simulink library "INT_ASDrf_SelectParameter"  (R2016b)
settings: Solver=VariableStepAuto  StartTime=0.0  StopTime=10.0  RelTol=1e-3
settings Model: Creator=lenovo  LastModifiedBy=lenovo

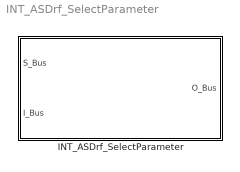
== system INT_ASDrf_SelectParameter ==
  INT_ASDrf_SelectParameter : Subsystem

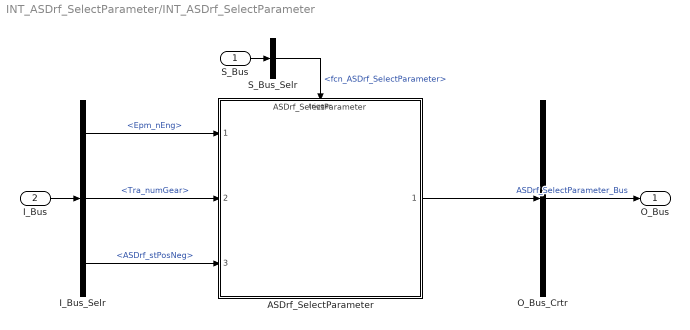
== system INT_ASDrf_SelectParameter/INT_ASDrf_SelectParameter ==
  S_Bus : Inport
  I_Bus : Inport  Port=2
  ASDrf_SelectParameter : ModelReference  ModelNameDialog=ASDrf_SelectParameter  SimulationMode=Normal  ModelReferenceVersion=1.11  TriggerPortName=function  TriggerPortTriggerType=function-call  TriggerPortStatesWhenEnabling=held
  I_Bus_Selr : BusSelector  OutputSignals=Epm_nEng,Tra_numGear,ASDrf_stPosNeg
  O_Bus_Crtr : BusCreator  Inputs=1
  S_Bus_Selr : BusSelector  OutputSignals=fcn_ASDrf_SelectParameter
  O_Bus : Outport
  wires:
  S_Bus_Selr/1 -> ASDrf_SelectParameter/Trigger  "<fcn_ASDrf_SelectParameter>"
  S_Bus/1 -> S_Bus_Selr/1
  I_Bus/1 -> I_Bus_Selr/1
  I_Bus_Selr/1 -> ASDrf_SelectParameter/1  "<Epm_nEng>"
  I_Bus_Selr/2 -> ASDrf_SelectParameter/2  "<Tra_numGear>"
  I_Bus_Selr/3 -> ASDrf_SelectParameter/3  "<ASDrf_stPosNeg>"
  O_Bus_Crtr/1 -> O_Bus/1  "ASDrf_SelectParameter_Bus"
  ASDrf_SelectParameter/1 -> O_Bus_Crtr/1
